simulink model "Animation_Try_2"  (R2025a)
settings: Solver=FixedStepAuto  StartTime=0.0  StopTime=500  FixedStep=0.01  RelTol=1e-3
undefined symbols (not defined in the file): DiscIntNeverNeededParam
libraries: aerolibanim x1, aerolibatmos2 x1, sharedutil x1
settings Model: Creator=shauryagupta  LastModifiedBy=shauryagupta

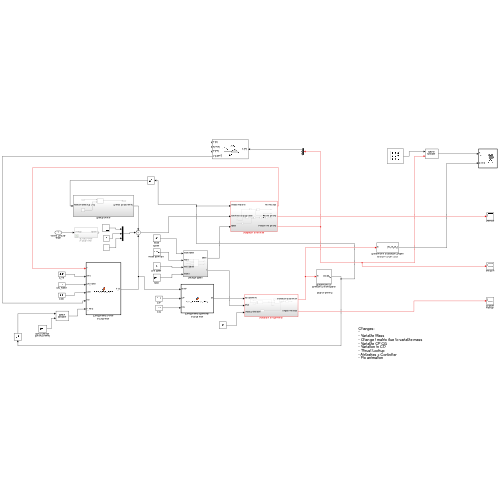
[thumbnail: Simulink's stored preview of the top-level diagram]
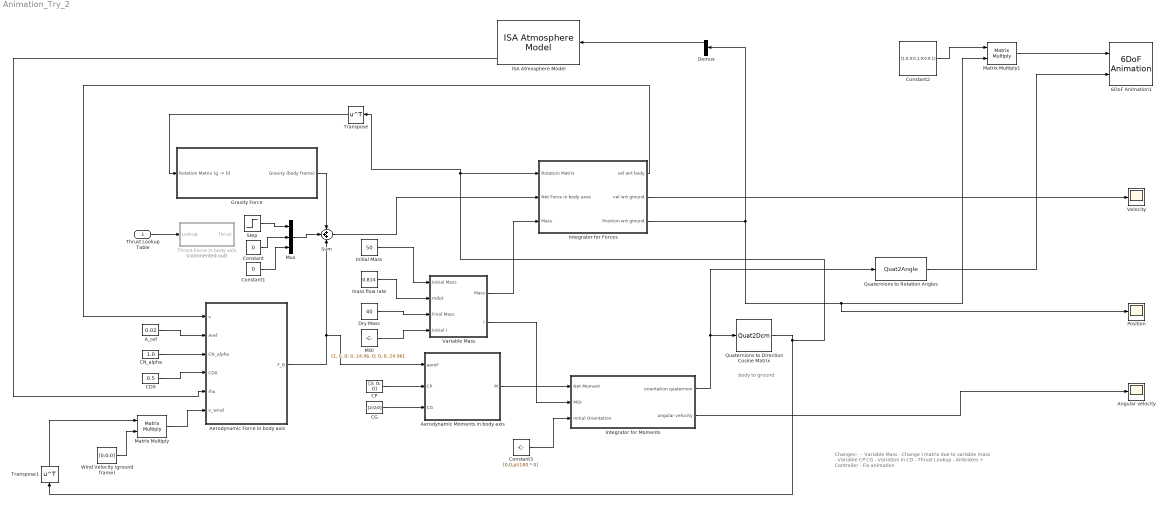
== system Animation_Try_2 ==
  note: Changes:
      | -
      | - Variable Mass
      | - Change I matrix due to variable mass
      | - Variable CP CG
      | - Variation in CD
      | - Thrust Lookup
      | - Airbrakes + Controller
      | - Fix animation
  note: body to ground
  Thrust Lookup Table : Inport
  6DoF Animation1 : aerolibanim/6DoF Animation  u1=[0 4000 -2000 2000 -5000 -3000]  u2=0.2  u3=100  u4=[4000 0 -5000]  u5=Fly alongside  u6=[2000 500 -3150]  u7=10  u8=on
  A_ref : Constant  Value=0.02
  Aerodynamic Force in body axis : MATLAB Function  TreatAsAtomicUnit=on
  Aerodynamic Moments in body axis : MATLAB Function  TreatAsAtomicUnit=on
  Angular velocity : Scope
      settings: ActiveDisplayYMinimum=-1  ActiveDisplayYMaximum=1  DataLoggingVariableName=ScopeData2
  CD0 : Constant  Value=0.5
  CG : Constant  Value=[2;0;0]  VectorParams1D=off
  CN_alpha : Constant  Value=1.0
  CP : Constant  Value=[3; 0; 0]
  Constant : Constant  Value=0
  Constant1 : Constant  Value=0
  Constant2 : Constant  Value=[1,0,0;0,1,0;0,0,1]
  Constant3 : Constant  Value=[0,0,pi/180 * 0]  VectorParams1D=off
  Demux : Demux  Outputs=3
  Dry Mass : Constant  Value=40
  Gravity Force : Subsystem
  ISA Atmosphere Model : aerolibatmos2/ISA Atmosphere Model  useExtended=off  action=None  custom=off  viscosityOut=off  g=9.80665  gamma=1.4  R=287.0531  L=0.0065  h_trop=11000  h_strat=20000  rho0=1.225  P0=101325  T0=288.15  h0=0  S=110.4  Tref=273.15  muref=1.716e-5
  Initial Mass : Constant  Value=50
  Integrator for Forces : Subsystem
  Integrator for Moments : Subsystem
  MOI : Constant  Value=[1, 0, 0; 0, 24.96, 0; 0, 0, 24.96]
  Matrix Multiply : Product  Multiplication=Matrix(*)
  Matrix Multiply1 : Product  Multiplication=Matrix(*)
  Mux : Mux  Inputs=3
  Position : Scope
      settings: ActiveDisplayYMinimum=-4325.8492002642852  ActiveDisplayYMaximum=38932.642802378577
  "Quaternions to Direction Cosine Matrix " : Quat2Dcm
  Quaternions to Rotation Angles : Quat2Angle  rotationOrder=XYZ
      settings: AttributesFormatString=Rotation Order: %<rotationOrder>
  Step : Step  Time=6.95  Before=250  After=0  SampleTime=0
  Sum : Sum  Inputs=+++
  "Thrust Force in body axis " : Subsystem  Commented=on
  Transpose : Math  Operator=transpose
  Transpose1 : Math  Operator=transpose
  Variable Mass : Subsystem
  Velocity : Scope
      settings: ActiveDisplayYMinimum=-41.710609905049544  ActiveDisplayYMaximum=375.39548914544594
  Wind Velocity (ground frame) : Constant  Value=[0;0;0]
  "mass flow rate " : Constant  Value=0.814
  wires:
  "Quaternions to Direction Cosine Matrix "/1 -> Transpose/1, Integrator for Forces/1(Rotation Matrix), Transpose1/1
  CP/1 -> Aerodynamic Moments in body axis/2(CP)
  Constant3/1 -> Integrator for Moments/3(Initial Orientation)
  Transpose/1 -> Gravity Force/1("Rotation Matrix (g -> b) ")
  Integrator for Forces/1(vel wrt body) -> Aerodynamic Force in body axis/1(v)
  Constant1/1 -> Mux/3
  Constant/1 -> Mux/2
  Mux/1 -> Sum/2
  Integrator for Moments/1(orientation quaternion) -> Quaternions to Rotation Angles/1, "Quaternions to Direction Cosine Matrix "/1
  Matrix Multiply/1 -> Aerodynamic Force in body axis/6(v_wind)
  ISA Atmosphere Model/4 -> Aerodynamic Force in body axis/5(rho)
  Constant2/1 -> Matrix Multiply1/1
  CG/1 -> Aerodynamic Moments in body axis/3(CG)
  Sum/1 -> Integrator for Forces/2("Net Force in body axes ")
  CN_alpha/1 -> Aerodynamic Force in body axis/3(CN_alpha)
  Integrator for Forces/2(vel wrt ground) -> Velocity/1
  A_ref/1 -> Aerodynamic Force in body axis/2(Aref)
  CD0/1 -> Aerodynamic Force in body axis/4(CD0)
  Transpose1/1 -> Matrix Multiply/1
  Integrator for Forces/3(Position wrt ground) -> Demux/1, Matrix Multiply1/2, Position/1
  Aerodynamic Force in body axis/1(F_B) -> Sum/3, Aerodynamic Moments in body axis/1(aeroF)
  Aerodynamic Moments in body axis/1(M) -> Integrator for Moments/1(Net Moment)
  Thrust Lookup Table/1 -> "Thrust Force in body axis "/1(Lookup)
  Matrix Multiply1/1 -> 6DoF Animation1/1
  Integrator for Moments/2(angular velocity) -> Angular velocity/1
  Demux/1 -> ISA Atmosphere Model/1
  Initial Mass/1 -> Variable Mass/1(Initial Mass)
  Gravity Force/1(Gravity (body frame)) -> Sum/1
  Wind Velocity (ground frame)/1 -> Matrix Multiply/2
  Quaternions to Rotation Angles/1 -> 6DoF Animation1/2
  Step/1 -> Mux/1
  "mass flow rate "/1 -> Variable Mass/2(mdot)
  Dry Mass/1 -> Variable Mass/3(Final Mass)
  Variable Mass/1(Mass) -> Integrator for Forces/3(Mass)
  Variable Mass/2(I) -> Integrator for Moments/2(MOI)
  MOI/1 -> Variable Mass/4(Initial I)

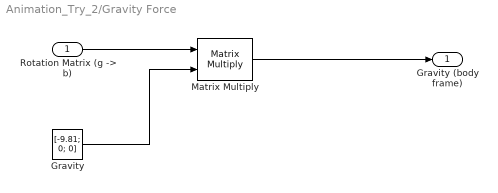
== system Animation_Try_2/Gravity Force ==
  "Rotation Matrix (g -> b) " : Inport
  Gravity : Constant  Value=[-9.81; 0; 0]
  Matrix Multiply : Product  Multiplication=Matrix(*)
  Gravity (body frame) : Outport
  wires:
  "Rotation Matrix (g -> b) "/1 -> Matrix Multiply/1
  Gravity/1 -> Matrix Multiply/2
  Matrix Multiply/1 -> Gravity (body frame)/1

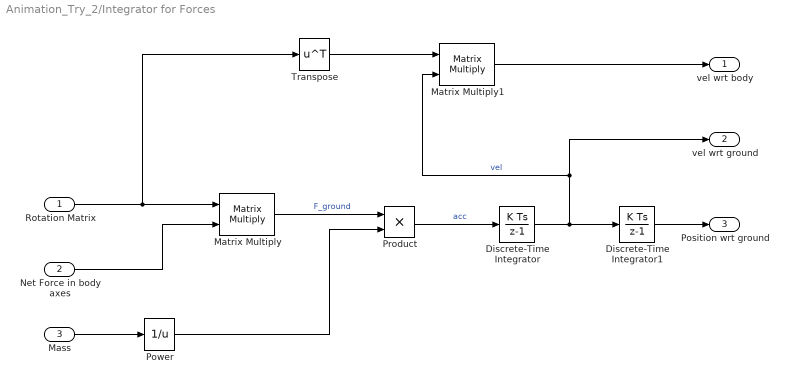
== system Animation_Try_2/Integrator for Forces ==
  Rotation Matrix : Inport
  "Net Force in body axes " : Inport  Port=2
  Mass : Inport  Port=3
  Discrete-Time Integrator : DiscreteIntegrator  SampleTime=-1  ICPrevOutput=DiscIntNeverNeededParam  ICPrevScaledInput=DiscIntNeverNeededParam
  Discrete-Time Integrator1 : DiscreteIntegrator  SampleTime=-1  ICPrevOutput=DiscIntNeverNeededParam  ICPrevScaledInput=DiscIntNeverNeededParam
  Matrix Multiply : Product  Multiplication=Matrix(*)
  Matrix Multiply1 : Product  Multiplication=Matrix(*)
  Power : Math  Operator=reciprocal
  Product : Product
  Transpose : Math  Operator=transpose
  vel wrt body : Outport
  vel wrt ground : Outport  Port=2
  Position wrt ground : Outport  Port=3
  wires:
  Rotation Matrix/1 -> Transpose/1, Matrix Multiply/1
  "Net Force in body axes "/1 -> Matrix Multiply/2
  Mass/1 -> Power/1
  Matrix Multiply/1 -> Product/1  "F_ground"
  Power/1 -> Product/2
  Product/1 -> Discrete-Time Integrator/1  "acc"
  Discrete-Time Integrator/1 -> Discrete-Time Integrator1/1, Matrix Multiply1/2, vel wrt ground/1  "vel"
  Discrete-Time Integrator1/1 -> Position wrt ground/1
  Transpose/1 -> Matrix Multiply1/1
  Matrix Multiply1/1 -> vel wrt body/1

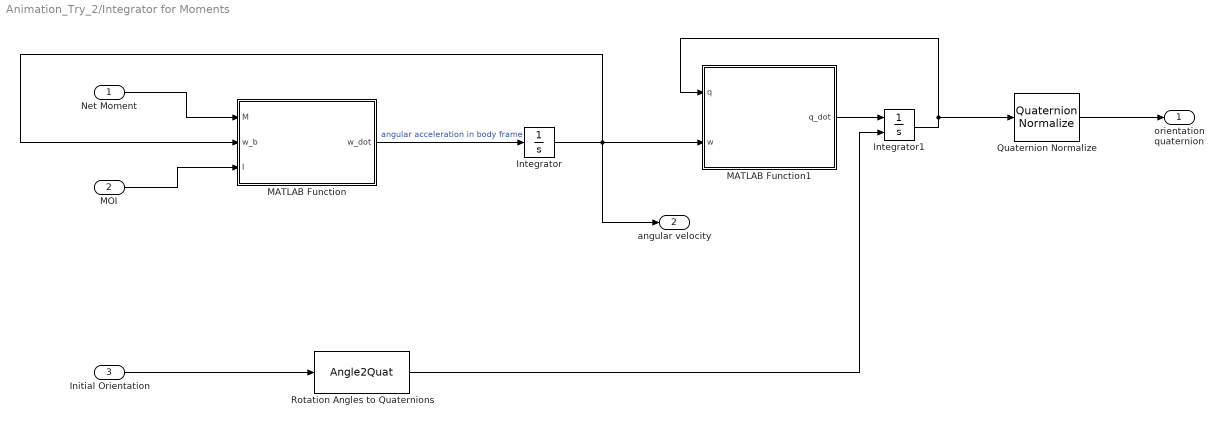
== system Animation_Try_2/Integrator for Moments ==
  Net Moment : Inport
  MOI : Inport  Port=2
  Initial Orientation : Inport  Port=3
  Integrator : Integrator  InitialCondition=[0; 0; 0]
  Integrator1 : Integrator  InitialConditionSource=external  InitialCondition=[1; 0; 0; 0]  ContinuousStateAttributes='orientation'
  MATLAB Function : MATLAB Function  TreatAsAtomicUnit=on
  MATLAB Function1 : MATLAB Function  TreatAsAtomicUnit=on
  Quaternion Normalize : sharedutil/Quaternion Normalize  aMode=aMode
  Rotation Angles to Quaternions : Angle2Quat  rotationOrder=XYZ
      settings: AttributesFormatString=Rotation Order: %<rotationOrder>
  orientation quaternion : Outport
  angular velocity : Outport  Port=2
  wires:
  Net Moment/1 -> MATLAB Function/1(M)
  MOI/1 -> MATLAB Function/3(I)
  Integrator/1 -> MATLAB Function/2(w_b), MATLAB Function1/2(w), angular velocity/1
  MATLAB Function/1(w_dot) -> Integrator/1  "angular acceleration in body frame"
  MATLAB Function1/1(q_dot) -> Integrator1/1
  Integrator1/1 -> MATLAB Function1/1(q), Quaternion Normalize/1
  Quaternion Normalize/1 -> orientation quaternion/1
  Rotation Angles to Quaternions/1 -> Integrator1/2
  Initial Orientation/1 -> Rotation Angles to Quaternions/1

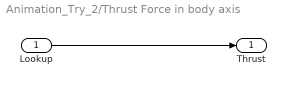
== system Animation_Try_2/Thrust Force in body axis  ==
  Lookup : Inport
  Thrust : Outport
  wires:
  Lookup/1 -> Thrust/1

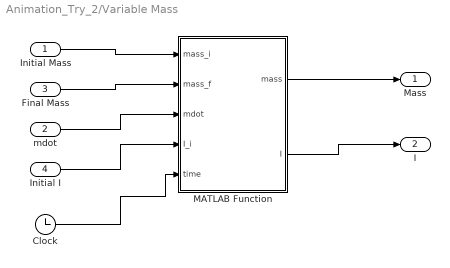
== system Animation_Try_2/Variable Mass ==
  Initial Mass : Inport
  mdot : Inport  Port=2
  Final Mass : Inport  Port=3
  Initial I : Inport  Port=4
  Clock : Clock
  MATLAB Function : MATLAB Function  TreatAsAtomicUnit=on
  Mass : Outport
  I : Outport  Port=2
  wires:
  Initial Mass/1 -> MATLAB Function/1(mass_i)
  mdot/1 -> MATLAB Function/3(mdot)
  Final Mass/1 -> MATLAB Function/2(mass_f)
  Initial I/1 -> MATLAB Function/4(I_i)
  Clock/1 -> MATLAB Function/5(time)
  MATLAB Function/2(I) -> I/1
  MATLAB Function/1(mass) -> Mass/1

== matlab function Animation_Try_2/Integrator for Moments/MATLAB Function ==
  data: M input; w_dot output; w_b input; I input
function w_dot = angular_vel(M, w_b, I)
%#codegen


angular_vel = I \ ( M - cross(w_b, I*w_b) );

w_dot = angular_vel;

if any(~isfinite(M))
    w_dot = [0;0;0];
    return
end

== matlab function Animation_Try_2/Aerodynamic Moments in body axis ==
  data: aeroF input; M output; CP input; CG input
function M = aero_moments_body(aeroF, CP, CG)
%#codegen
% CP, CG, Fb -> 3 X 1 vectors


r = CP - CG;

if norm(aeroF) < 1e-3
    M = [0; 0; 0];
else
    M = cross(r, aeroF);

end

== matlab function Animation_Try_2/Integrator for Moments/MATLAB Function1 ==
  data: q input; q_dot output; w input
function q_dot = quat_dot_from_omega(q, w)
% Inputs:
%   q : 4x1 quaternion [q0; q1; q2; q3]
%   w : 3x1 angular velocity [wx; wy; wz] (rad/s)
%
% Output:
%   q_dot : 4x1 quaternion derivative

wx = w(1);
wy = w(2);
wz = w(3);

Omega = [  0  -wx -wy -wz;
           wx   0  -wz  wy;
           wy   wz  0  -wx;
           wz  -wy  wx  0 ];

q_dot = 0.5 * Omega * q;
end

== matlab function Animation_Try_2/Variable Mass/MATLAB Function ==
  data: mass_i input; mass output; mass_f input; mdot input; I_i input; time input; I output
function [mass,I] = variable_mass(mass_i, mass_f, mdot, I_i, time)


t_burn = (mass_i - mass_f)/mdot;

if time <= t_burn
    mass = mass_i - mdot*time;
else
    mass = mass_f;
end
   
I = I_i * mass / mass_i;

== matlab function Animation_Try_2/Aerodynamic Force in body axis ==
  data: v input; F_B output; Aref input; CN_alpha input; CD0 input; rho input; v_wind input
function F_B = aero_forces_body(v, Aref, CN_alpha, CD0, rho, v_wind)
% ----------------------------------------------------
% Computes total aerodynamic force in BODY frame
%
% Inputs:
% vB   : 3x1 velocity vector in body frame [m/s]
% rho  : air density [kg/m^3]
% Aref : reference area [m^2]
% CN   : normal force coefficient
% CD   : drag coefficient
%
% Output:
% F_B  : 3x1 aerodynamic force vector in body frame [N]
% ----------------------------------------------------

% Unpack velocity

vB = v - v_wind;

vx = vB(1);
vy = vB(2);
vz = vB(3);


V = norm(vB);

% Guard against zero velocity
if V < 1e-3
    F_B = [0; 0; 0];
    return
end

% Dynamic pressure
q = 0.5 * rho * V^2;

% -------------------------
% Drag force (opposite wind)
% -------------------------
drag_dir = -vB / V;   % unit vector opposite rocket velocity
F_normal = -CN_alpha * q * Aref * [0; vB(2); vB(3)] / V;
CD = CD0;
F_drag = CD * q * Aref * drag_dir;


% -------------------------
% Total aerodynamic force
% -------------------------
F_B = F_drag + F_normal;

end
